simulink model "EspacioEstados"  (R2019a)
settings: Solver=VariableStepAuto  StartTime=0.0  StopTime=8  RelTol=1e-3
values from neighbouring files (symbols this model uses):
  A = [0        1               0 ... (first row only)    [MatricesEspaciodeEstados.m]
  B = 0.2    [ConvertirEspacioDeEstados.m]    (also in KuTu.m; MatricesEspaciodeEstados.m = [0; MotorPorArmadura.m; sIntonizacionPID.m)
  C = pid(Kp, Ki, Kd)    [KuTu.m]    (also in MatricesEspaciodeEstados.m = [0 1 0]; sIntonizacionPID.m)
  D = 0    [MatricesEspaciodeEstados.m]
  Va = 5    [MatricesEspaciodeEstados.m]
libraries: simulink x1
settings Model: Creator=MSI GAMER  LastModifiedBy=MSI GAMER

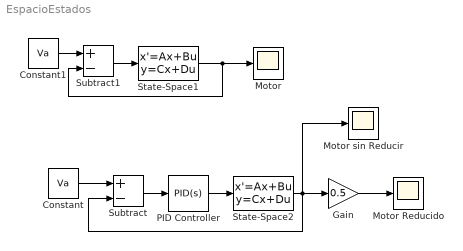
== system EspacioEstados ==
  Constant : Constant  Value=Va
  Constant1 : Constant  Value=Va
  Gain : Gain  Gain=0.5
  Motor : Scope
  Motor Reducido : Scope
  Motor sin Reducir : Scope
  PID Controller : simulink/Continuous/PID Controller  Controller=PID  Form=Parallel  TimeDomain=Continuous-time  SampleTime=-1  IntegratorMethod=Forward Euler  FilterMethod=Forward Euler  ControllerParametersSource=internal  P=49.95  I=76.93  D=7.87  UseFilter=on  N=100  TunerSelectOption=Transfer Function Based (PID Tuner App)  InitialConditionSource=internal  InitialConditionForIntegrator=0  InitialConditionForFilter=0  DifferentiatorICPrevScaledInput=0  ExternalReset=none  TrackingMode=off  Kt=1  LimitOutput=off  UpperSaturationLimit=inf  LowerSaturationLimit=-inf  LinearizeAsGain=on  AntiWindupMode=none  Kb=1  POutMin=[]  POutMax=[]  IOutMin=[]  IOutMax=[]  DOutMin=[]  DOutMax=[]  NOutMin=[]  NOutMax=[]  SumOutMin=[]  SumOutMax=[]  SaturationOutMin=[]  SaturationOutMax=[]  PParamMin=[]  PParamMax=[]  IParamMin=[]  IParamMax=[]  DParamMin=[]  DParamMax=[]  NParamMin=[]  NParamMax=[]  KbParamMin=[]  KbParamMax=[]  KtParamMin=[]  KtParamMax=[]  KbOutMin=[]  KbOutMax=[]  KtOutMin=[]  KtOutMax=[]  IntegratorOutMin=[]  IntegratorOutMax=[]  FilterOutMin=[]  FilterOutMax=[]  SumI1OutMin=[]  SumI1OutMax=[]  SumI2OutMin=[]  SumI2OutMax=[]  SumI3OutMin=[]  SumI3OutMax=[]  SumI4OutMin=[]  SumI4OutMax=[]  SumDOutMin=[]  SumDOutMax=[]  DifferentiatorOutMin=[]  DifferentiatorOutMax=[]  FilterDiffOutCoefMin=[]  FilterDiffOutCoefMax=[]  ReciprocalOutMin=[]  ReciprocalOutMax=[]  SumDenOutMin=[]  SumDenOutMax=[]  SumNumOutMin=[]  SumNumOutMax=[]  DivideOutMin=[]  DivideOutMax=[]  IntegratorContinuousStateAttributes=''  IntegratorStateMustResolveToSignalObject=off  IntegratorRTWStateStorageClass=Auto  FilterContinuousStateAttributes=''  FilterStateMustResolveToSignalObject=off  FilterRTWStateStorageClass=Auto  ParallelPVariant=InternalParameters  IdealPVariant=Disabled  IVariant=InternalParameters  DVariant=InternalParameters  IntegratorVariant=Continuous  SatVariant=Disabled  AWVariant=Passthrough  PCopyVariant=Disabled  TRVariant=Disabled  FdbkBlocksVariant=Forward  IdealPFdbkVariant=Disabled  SatFdbkVariant=Disabled  DerivativeFilterVariant=ContFilter  NVariant=InternalParameters  NCopyVariant=Disabled  FilterICVariant=InternalICsFilter  IntegratorICVariant=InternalICs  ExternalResetVariant=Disabled  TRSumVariant=Passthrough  SumFdbkVariant=Disabled  SumVariant=Sum_PID
  State-Space1 : StateSpace  A=A  B=B  C=C  D=D  InitialCondition=0  ContinuousStateAttributes='estados'
  State-Space2 : StateSpace  A=A  B=B  C=C  D=D  InitialCondition=0  ContinuousStateAttributes='estados'
  Subtract : Sum  Inputs=+-
  Subtract1 : Sum  Inputs=+-
  wires:
  Subtract/1 -> PID Controller/1
  State-Space2/1 -> Motor sin Reducir/1, Subtract/2, Gain/1
  Gain/1 -> Motor Reducido/1
  PID Controller/1 -> State-Space2/1
  Constant/1 -> Subtract/1
  Subtract1/1 -> State-Space1/1
  Constant1/1 -> Subtract1/1
  State-Space1/1 -> Motor/1, Subtract1/2
